simulink model "SCo3"  (Simulink 8.5)
settings: Solver=ode23t  SolverMode=SingleTasking  StartTime=0.0  StopTime=0.1  RelTol=1e-3  AbsTol=1e-3
libraries: powerlib x41, powerlib_extras x9
settings Model: Creator=azadpour  LastModifiedBy=PC  ExtModeTrigMode=oneshot  ExtModeArmWhenConnect=off  ExtModeAutoUpdateStatusClock=off
settings DataIOCC: LimitDataPoints=off
settings OptimizationCC: BlockReduction=off  BooleanDataType=off  InitFltsAndDblsToZero=on
settings DebuggingCC: SaveWithParameterizedLinksMsg=none  SignalResolutionControl=TryResolveAllWithWarning  InheritedTsInSrcMsg=none  MultiTaskDSMMsg=warning  MultiTaskCondExecSysMsg=none  FcnCallInpInsideContextMsg=UseLocalSettings  StrictBusMsg=None
settings HardwareCC: TargetUnknown=on
settings RTWCC: TemplateMakefile=grt_vc.tmf
settings GRTTargetCC: TargetFcnLib=ansi_tfl_tmw.mat

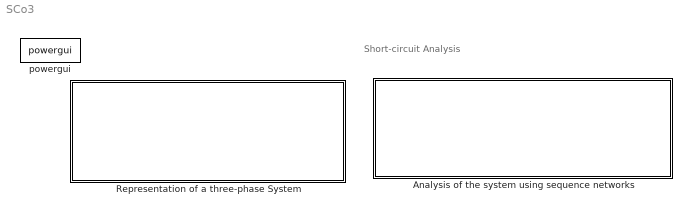
== system SCo3 ==
  note: Short-circuit Analysis
  Analysis of the system using sequence networks : Subsystem
      mask Display: disp('Analysis of the system using sequence networks')
  Representation of a three-phase System : Subsystem
      mask Display: disp('Representaton of a three-phase System')
  powergui : powerlib/powergui  SimulationMode=Continuous  SolverType=Tustin/Backward Euler (TBE)  SampleTime=0  frequency=60  SPID=off  DisableSnubberDevices=off  DisableRonSwitches=off  DisableVfSwitches=off  SwTol=0  DisplayEquations=off  Interpol=off  methode=off  Ts=0  FunctionMessages=off  echomessages=off  HookPort=off  EnableUseOfTLC=off  x0status=blocks  frequencyindice=0  Pbase=100e6  ErrMax=1e-4  Iterations=50  UnitsV=kV  UnitsW=MW  buscounter=0  RestoreLinks=warning  ResistiveCurrentMeasurement=off  Frange=[0:2:500]  Ylog=off  Xlog=on  ShowGrid=off  save=off  variable=ZData  structure=0  ZoomFFT=on  StartTime=0.0  cycles=1  DisplayStyle=1  fundamental=60  FreqAxis=off  MaxFrequency=1000  frequencyindicesteady=1  RmsSteady=1  display=off

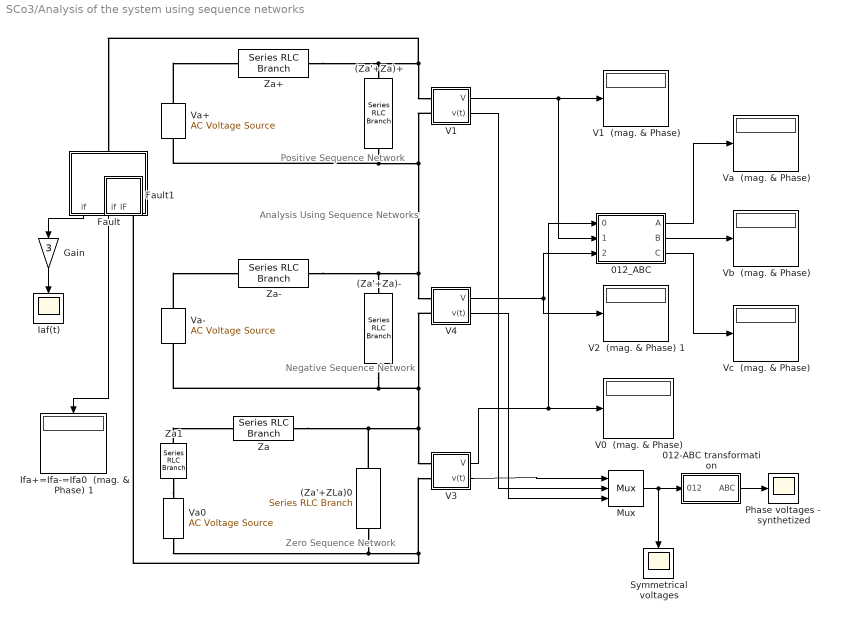
== system SCo3/Analysis of the system using sequence networks ==
  note: Positive Sequence Network
  note: Zero Sequence Network
  note: Negative Sequence Network
  note: Analysis Using
      | Sequence Networks
  (Za'+ZLa)0 : powerlib/Elements/Series RLC Branch  LConnTagsString=__new0  RConnTagsString=__new0  BranchType=RL  Resistance=0.01+0.72  Inductance=(0.05+0.54)/(2*pi*60)  SetiL0=off  InitialCurrent=0  Capacitance=1.0  Setx0=off  InitialVoltage=0  Measurements=None
  (Za'+Za)+ : powerlib/Elements/Series RLC Branch  LConnTagsString=__new0  RConnTagsString=__new0  BranchType=RL  Resistance=0.01+0.72  Inductance=(0.05+0.54)/(2*pi*60)  SetiL0=off  InitialCurrent=0  Capacitance=1.0  Setx0=off  InitialVoltage=0  Measurements=None
  (Za'+Za)- : powerlib/Elements/Series RLC Branch  LConnTagsString=__new0  RConnTagsString=__new0  BranchType=RL  Resistance=0.01+0.72  Inductance=(0.05+0.54)/(2*pi*60)  SetiL0=off  InitialCurrent=0  Capacitance=1.0  Setx0=off  InitialVoltage=0  Measurements=None
  012-ABC transformation : Subsystem
  012_ABC : Subsystem
      mask init:
      | a=cos(120*pi/180)+i*sin(120*pi/180);
      | A=[1 1 1; 1 a^2 a; 1 a a^2];
      mask Display: disp('012_ABC');
  Fault : Subsystem  mask{RF=3*0.5, time=(2.25)/60}
      mask prompts: RF "Resistance [ohm]"; time "Time [sec]"
      mask Display: plot(0,0,100,100,[40,40,57,35,51],[20,5,73,48,95],[40,51],[5,20])
  Fault1 : Subsystem  mask{RF=3*0.5, time=(2.25)/60}
      mask prompts: RF "Resistance [ohm]"; time "Time [sec]"
      mask Display: plot(0,0,100,100,[40,40,57,35,51],[20,5,73,48,95],[40,51],[5,20])
  Gain : Gain  Gain=3  SaturateOnIntegerOverflow=on  OutDataTypeStr=Inherit: Same as input  ParamDataTypeStr=Inherit: Same as input
  Iaf(t) : Scope
      settings: TickLabels=on  TimeRange=0.1  YMin=-1.5  YMax=1.5
  Ifa+=Ifa-=Ifa0  (mag. & Phase) 1 : Display
  Mux : Mux  Inputs=3
  Phase voltages -  synthetized : Scope
      settings: TickLabels=on  TimeRange=0.1  YMin=-1.3  YMax=1.3
  Symmetrical voltages : Scope
      settings: TickLabels=on  TimeRange=0.05  YMin=-1.05  YMax=1.05
  "V0  (mag. & Phase) " : Display
  V1 : Subsystem
  "V1  (mag. & Phase) " : Display
  V2  (mag. & Phase) 1 : Display
  V3 : Subsystem
  V4 : Subsystem
  "Va  (mag. & Phase) " : Display
  Va+ : powerlib/Electrical Sources/AC Voltage Source  Amplitude=1  Phase=0  Frequency=60  SampleTime=0  Measurements=None
  Va- : powerlib/Electrical Sources/AC Voltage Source  Amplitude=0  Phase=0  Frequency=60  SampleTime=0  Measurements=None
  Va0 : powerlib/Electrical Sources/AC Voltage Source  Amplitude=0  Phase=0  Frequency=60  SampleTime=0  Measurements=None
  "Vb  (mag. & Phase) " : Display
  "Vc  (mag. & Phase) " : Display
  Za : powerlib/Elements/Series RLC Branch  LConnTagsString=__new0  RConnTagsString=__new0  BranchType=RL  Resistance=0.01  Inductance=0.05/(2*pi*60)  SetiL0=off  InitialCurrent=0  Capacitance=1.0  Setx0=off  InitialVoltage=0  Measurements=None
  Za+ : powerlib/Elements/Series RLC Branch  LConnTagsString=__new0  RConnTagsString=__new0  BranchType=RL  Resistance=0.01  Inductance=0.05/(2*pi*60)  SetiL0=off  InitialCurrent=0  Capacitance=1.0  Setx0=off  InitialVoltage=0  Measurements=None
  Za- : powerlib/Elements/Series RLC Branch  LConnTagsString=__new0  RConnTagsString=__new0  BranchType=RL  Resistance=0.01  Inductance=0.05/(2*pi*60)  SetiL0=off  InitialCurrent=0  Capacitance=1.0  Setx0=off  InitialVoltage=0  Measurements=None
  Za1 : powerlib/Elements/Series RLC Branch  LConnTagsString=__new0  RConnTagsString=__new0  BranchType=Open circuit  Resistance=1  Inductance=1.0  SetiL0=off  InitialCurrent=0  Capacitance=1.0  Setx0=off  InitialVoltage=0  Measurements=None
  wires:
  Gain/1 -> Iaf(t)/1
  Fault/1(if) -> Gain/1
  Fault/2(IF) -> Ifa+=Ifa-=Ifa0  (mag. & Phase) 1/1
  012-ABC transformation/1(ABC) -> Phase voltages -  synthetized/1
  V1/2(v(t)) -> Mux/2
  V4/2(v(t)) -> Mux/3
  V3/2(v(t)) -> Mux/1
  012_ABC/1(A) -> "Va  (mag. & Phase) "/1
  012_ABC/2(B) -> "Vb  (mag. & Phase) "/1
  012_ABC/3(C) -> "Vc  (mag. & Phase) "/1
  V3/1(V) -> 012_ABC/1(0), "V0  (mag. & Phase) "/1
  V4/1(V) -> 012_ABC/3(2), V2  (mag. & Phase) 1/1
  V1/1(V) -> "V1  (mag. & Phase) "/1, 012_ABC/2(1)
  Mux/1 -> 012-ABC transformation/1(012), Symmetrical voltages/1
  connections:
  Va+/RConn1 -- Za+/LConn1
  Za-/RConn1 -- V1/LConn2 -- Va+/LConn1 -- (Za'+Za)+/RConn1 -- V4/LConn1 -- (Za'+Za)-/LConn1
  (Za'+ZLa)0/RConn1 -- Fault/RConn1 -- V3/LConn2 -- Va0/LConn1
  (Za'+ZLa)0/LConn1 -- V4/LConn2 -- Va-/LConn1 -- (Za'+Za)-/RConn1 -- V3/LConn1 -- Za/RConn1
  Va-/RConn1 -- Za-/LConn1
  Za+/RConn1 -- (Za'+Za)+/LConn1 -- V1/LConn1 -- Fault/LConn1
  Za1/RConn1 -- Va0/RConn1
  Za1/LConn1 -- Za/LConn1

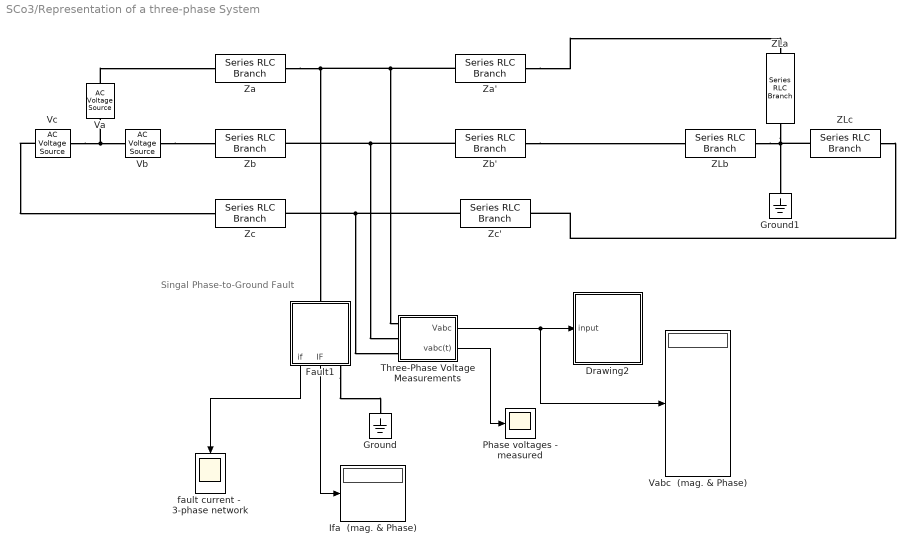
== system SCo3/Representation of a three-phase System ==
  note: Singal Phase-to-Ground Fault
  Drawing2 : Subsystem  mask(ABC and 012 Phasor Display){Bactive=off}
      mask prompts: Bactive "Block active"
      mask init:
      | global count;
      | count=0;
      mask Display: disp('Display \nabc \nand \n012\nphasors');
  Fault1 : Subsystem  mask{RF=0.5, time=(2.25)/60}
      mask prompts: RF "Resistance [ohm]"; time "Time [sec]"
      mask Display: plot(0,0,100,100,[40,40,57,35,51],[20,5,73,48,95],[40,51],[5,20])
  Ground : powerlib/Elements/Ground  LConnTagsString=a
  Ground1 : powerlib/Elements/Ground  LConnTagsString=a
  Ifa  (mag. & Phase) : Display
  Phase voltages - measured : Scope
      settings: TickLabels=on  TimeRange=0.1  YMin=-1.3  YMax=1.3
  Three-Phase Voltage Measurements : Subsystem
  Va : powerlib/Electrical Sources/AC Voltage Source  Amplitude=1  Phase=0  Frequency=60  SampleTime=0  Measurements=None
  Vabc  (mag. & Phase) : Display
  Vb : powerlib/Electrical Sources/AC Voltage Source  Amplitude=1  Phase=-120  Frequency=60  SampleTime=0  Measurements=None
  Vc : powerlib/Electrical Sources/AC Voltage Source  Amplitude=1  Phase=120  Frequency=60  SampleTime=0  Measurements=None
  ZLa : powerlib/Elements/Series RLC Branch  LConnTagsString=__new0  RConnTagsString=__new0  BranchType=RL  Resistance=0.72  Inductance=0.54/(2*pi*60)  SetiL0=off  InitialCurrent=0  Capacitance=1.0  Setx0=off  InitialVoltage=0  Measurements=None
  ZLb : powerlib/Elements/Series RLC Branch  LConnTagsString=__new0  RConnTagsString=__new0  BranchType=RL  Resistance=0.72  Inductance=0.54/(2*pi*60)  SetiL0=off  InitialCurrent=0  Capacitance=1.0  Setx0=off  InitialVoltage=0  Measurements=None
  ZLc : powerlib/Elements/Series RLC Branch  LConnTagsString=__new0  RConnTagsString=__new0  BranchType=RL  Resistance=0.72  Inductance=0.54/(2*pi*60)  SetiL0=off  InitialCurrent=0  Capacitance=1.0  Setx0=off  InitialVoltage=0  Measurements=None
  Za : powerlib/Elements/Series RLC Branch  LConnTagsString=__new0  RConnTagsString=__new0  BranchType=RL  Resistance=0.01  Inductance=0.05/(2*pi*60)  SetiL0=off  InitialCurrent=0  Capacitance=1.0  Setx0=off  InitialVoltage=0  Measurements=None
  Za' : powerlib/Elements/Series RLC Branch  LConnTagsString=__new0  RConnTagsString=__new0  BranchType=RL  Resistance=0.01  Inductance=0.05/(2*pi*60)  SetiL0=off  InitialCurrent=0  Capacitance=1.0  Setx0=off  InitialVoltage=0  Measurements=None
  Zb : powerlib/Elements/Series RLC Branch  LConnTagsString=__new0  RConnTagsString=__new0  BranchType=RL  Resistance=0.01  Inductance=0.05/(2*pi*60)  SetiL0=off  InitialCurrent=0  Capacitance=1.0  Setx0=off  InitialVoltage=0  Measurements=None
  Zb' : powerlib/Elements/Series RLC Branch  LConnTagsString=__new0  RConnTagsString=__new0  BranchType=RL  Resistance=0.01  Inductance=0.05/(2*pi*60)  SetiL0=off  InitialCurrent=0  Capacitance=1.0  Setx0=off  InitialVoltage=0  Measurements=None
  Zc : powerlib/Elements/Series RLC Branch  LConnTagsString=__new0  RConnTagsString=__new0  BranchType=RL  Resistance=0.01  Inductance=0.05/(2*pi*60)  SetiL0=off  InitialCurrent=0  Capacitance=1.0  Setx0=off  InitialVoltage=0  Measurements=None
  Zc' : powerlib/Elements/Series RLC Branch  LConnTagsString=__new0  RConnTagsString=__new0  BranchType=RL  Resistance=0.01  Inductance=0.05/(2*pi*60)  SetiL0=off  InitialCurrent=0  Capacitance=1.0  Setx0=off  InitialVoltage=0  Measurements=None
  fault current -  3-phase network : Scope
      settings: TickLabels=on  TimeRange=0.1  YMin=-1.5  YMax=1.5
  wires:
  Three-Phase Voltage Measurements/2(vabc(t)) -> Phase voltages - measured/1
  Three-Phase Voltage Measurements/1(Vabc) -> Drawing2/1(input), Vabc  (mag. & Phase)/1
  Fault1/1(if) -> fault current -  3-phase network/1
  Fault1/2(IF) -> Ifa  (mag. & Phase)/1
  connections:
  Vc/LConn1 -- Vb/LConn1 -- Va/LConn1
  Va/RConn1 -- Za/LConn1
  Vb/RConn1 -- Zb/LConn1
  Vc/RConn1 -- Zc/LConn1
  Za'/LConn1 -- Za/RConn1 -- Fault1/LConn1 -- Three-Phase Voltage Measurements/LConn1
  Zb'/LConn1 -- Zb/RConn1 -- Three-Phase Voltage Measurements/LConn2
  Zc'/LConn1 -- Zc/RConn1 -- Three-Phase Voltage Measurements/LConn3
  Fault1/RConn1 -- Ground/LConn1
  ZLa/RConn1 -- Ground1/LConn1 -- ZLc/RConn1 -- ZLb/RConn1
  Za'/RConn1 -- ZLa/LConn1
  Zb'/RConn1 -- ZLb/LConn1
  ZLc/LConn1 -- Zc'/RConn1

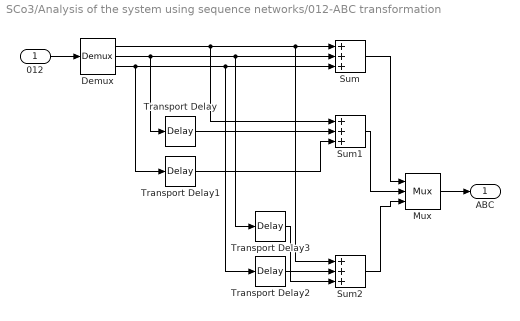
== system SCo3/Analysis of the system using sequence networks/012-ABC transformation ==
  012 : Inport
  Demux : Demux  Outputs=3
  Mux : Mux  Inputs=3
  Sum : Sum  Inputs=+++  SaturateOnIntegerOverflow=on  InputSameDT=on  OutDataTypeStr=Inherit: Same as first input
  Sum1 : Sum  Inputs=+++  SaturateOnIntegerOverflow=on  InputSameDT=on  OutDataTypeStr=Inherit: Same as first input
  Sum2 : Sum  Inputs=+++  SaturateOnIntegerOverflow=on  InputSameDT=on  OutDataTypeStr=Inherit: Same as first input
  Transport Delay : TransportDelay  DelayTime=1/(3*60)
  Transport Delay1 : TransportDelay  DelayTime=2/(3*60)
  Transport Delay2 : TransportDelay  DelayTime=1/(3*60)
  Transport Delay3 : TransportDelay  DelayTime=2/(3*60)
  ABC : Outport  InitialOutput=0
  wires:
  Transport Delay3/1 -> Sum2/2
  Transport Delay2/1 -> Sum2/3
  Transport Delay1/1 -> Sum1/3
  Transport Delay/1 -> Sum1/2
  Demux/1 -> Sum2/1, Sum/1, Sum1/1
  Demux/3 -> Transport Delay2/1, Sum/3, Transport Delay1/1
  Demux/2 -> Transport Delay3/1, Sum/2, Transport Delay/1
  Sum2/1 -> Mux/3
  Mux/1 -> ABC/1
  Sum/1 -> Mux/1
  Sum1/1 -> Mux/2
  012/1 -> Demux/1

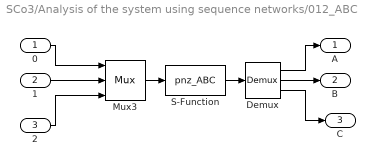
== system SCo3/Analysis of the system using sequence networks/012_ABC ==
  0 : Inport
  1 : Inport  Port=2
  2 : Inport  Port=3
  Demux : Demux  Outputs=3
  Mux3 : Mux  Inputs=3
  S-Function : S-Function  FunctionName=pnz_ABC  Parameters=A
  A : Outport  InitialOutput=0
  B : Outport  Port=2  InitialOutput=0
  C : Outport  Port=3  InitialOutput=0
  wires:
  Mux3/1 -> S-Function/1
  0/1 -> Mux3/1
  1/1 -> Mux3/2
  2/1 -> Mux3/3
  S-Function/1 -> Demux/1
  Demux/1 -> A/1
  Demux/2 -> B/1
  Demux/3 -> C/1

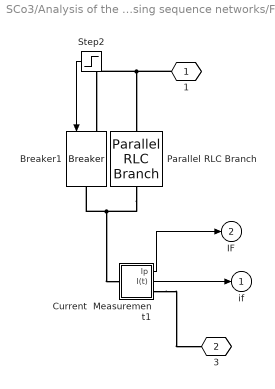
== system SCo3/Analysis of the system using sequence networks/Fault ==
  Breaker1 : powerlib/Elements/Breaker  InitialState=0  SwitchingTimes="[ 1/60  5/60 ]"  External=on  BreakerResistance=RF  SnubberResistance=1e6  SnubberCapacitance=inf  Measurements=None  MoreParameters=off  NoBreakLoop=off
  Current  Measurement1 : Subsystem
  Parallel RLC Branch : powerlib/Elements/Parallel RLC Branch  LConnTagsString=a  RConnTagsString=__new0  BranchType=R  Resistance=1e3  Inductance=1.0  SetiL0=off  InitialCurrent=0  Capacitance=1.0  Setx0=off  InitialVoltage=0  Measurements=None
  Step2 : Step  Time=time
  1 : PMIOPort  Tag=PMCPort  Port=1  Side=Left
  3 : PMIOPort  Tag=PMCPort  Port=2  Side=Right
  if : Outport  InitialOutput=0
  IF : Outport  Port=2  InitialOutput=0
  wires:
  Step2/1 -> Breaker1/1
  Current  Measurement1/2(I(t)) -> if/1
  Current  Measurement1/1(Ip) -> IF/1
  connections:
  1/RConn1 -- Breaker1/LConn1 -- Parallel RLC Branch/LConn1
  Parallel RLC Branch/RConn1 -- Breaker1/RConn1 -- Current  Measurement1/LConn1
  Current  Measurement1/RConn1 -- 3/RConn1

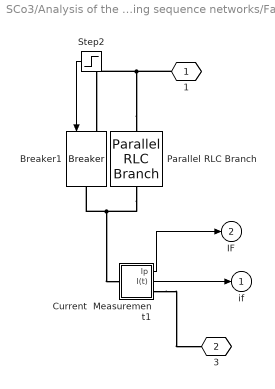
== system SCo3/Analysis of the system using sequence networks/Fault1 ==
  Breaker1 : powerlib/Elements/Breaker  InitialState=0  SwitchingTimes="[ 1/60  5/60 ]"  External=on  BreakerResistance=RF  SnubberResistance=1e6  SnubberCapacitance=inf  Measurements=None  MoreParameters=off  NoBreakLoop=off
  Current  Measurement1 : Subsystem
  Parallel RLC Branch : powerlib/Elements/Parallel RLC Branch  LConnTagsString=a  RConnTagsString=__new0  BranchType=R  Resistance=1e3  Inductance=1.0  SetiL0=off  InitialCurrent=0  Capacitance=1.0  Setx0=off  InitialVoltage=0  Measurements=None
  Step2 : Step  Time=time
  1 : PMIOPort  Tag=PMCPort  Port=1  Side=Left
  3 : PMIOPort  Tag=PMCPort  Port=2  Side=Right
  if : Outport  InitialOutput=0
  IF : Outport  Port=2  InitialOutput=0
  wires:
  Current  Measurement1/1(Ip) -> IF/1
  Current  Measurement1/2(I(t)) -> if/1
  Step2/1 -> Breaker1/1
  connections:
  Current  Measurement1/RConn1 -- 3/RConn1
  Current  Measurement1/LConn1 -- Breaker1/RConn1 -- Parallel RLC Branch/RConn1
  Parallel RLC Branch/LConn1 -- Breaker1/LConn1 -- 1/RConn1

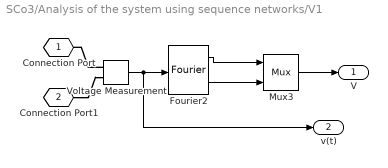
== system SCo3/Analysis of the system using sequence networks/V1 ==
  Fourier2 : powerlib_extras/Measurements/Fourier  f1=60  n=1
  Mux3 : Mux  Inputs=2
  Voltage Measurement : powerlib/Measurements/Voltage Measurement  PhasorSimulation=off  OutputType=Complex  PSBequivalent=0
  Connection Port : PMIOPort  Tag=PMCPort  Port=1  Side=Left
  Connection Port1 : PMIOPort  Tag=PMCPort  Port=2  Side=Left
  V : Outport  InitialOutput=0
  v(t) : Outport  Port=2  InitialOutput=0
  wires:
  Fourier2/1 -> Mux3/1
  Fourier2/2 -> Mux3/2
  Mux3/1 -> V/1
  Voltage Measurement/1 -> Fourier2/1, v(t)/1
  connections:
  Voltage Measurement/LConn1 -- Connection Port/RConn1
  Connection Port1/RConn1 -- Voltage Measurement/LConn2

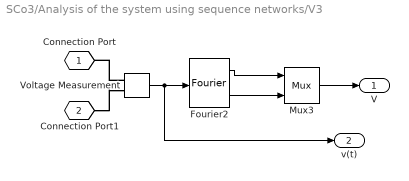
== system SCo3/Analysis of the system using sequence networks/V3 ==
  Fourier2 : powerlib_extras/Measurements/Fourier  f1=60  n=1
  Mux3 : Mux  Inputs=2
  Voltage Measurement : powerlib/Measurements/Voltage Measurement  PhasorSimulation=off  OutputType=Complex  PSBequivalent=0
  Connection Port : PMIOPort  Tag=PMCPort  Port=1  Side=Left
  Connection Port1 : PMIOPort  Tag=PMCPort  Port=2  Side=Left
  V : Outport  InitialOutput=0
  v(t) : Outport  Port=2  InitialOutput=0
  wires:
  Voltage Measurement/1 -> v(t)/1, Fourier2/1
  Mux3/1 -> V/1
  Fourier2/2 -> Mux3/2
  Fourier2/1 -> Mux3/1
  connections:
  Connection Port1/RConn1 -- Voltage Measurement/LConn2
  Voltage Measurement/LConn1 -- Connection Port/RConn1

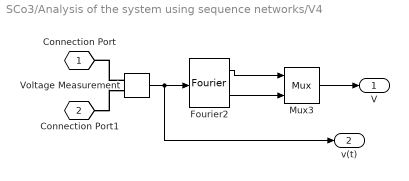
== system SCo3/Analysis of the system using sequence networks/V4 ==
  Fourier2 : powerlib_extras/Measurements/Fourier  f1=60  n=1
  Mux3 : Mux  Inputs=2
  Voltage Measurement : powerlib/Measurements/Voltage Measurement  PhasorSimulation=off  OutputType=Complex  PSBequivalent=0
  Connection Port : PMIOPort  Tag=PMCPort  Port=1  Side=Left
  Connection Port1 : PMIOPort  Tag=PMCPort  Port=2  Side=Left
  V : Outport  InitialOutput=0
  v(t) : Outport  Port=2  InitialOutput=0
  wires:
  Voltage Measurement/1 -> v(t)/1, Fourier2/1
  Mux3/1 -> V/1
  Fourier2/2 -> Mux3/2
  Fourier2/1 -> Mux3/1
  connections:
  Connection Port1/RConn1 -- Voltage Measurement/LConn2
  Voltage Measurement/LConn1 -- Connection Port/RConn1

== system SCo3/Representation of a three-phase System/Drawing2 ==
  input : Inport
  S-Function : S-Function  FunctionName=phdraw1c  Parameters=Bactive
  wires:
  input/1 -> S-Function/1

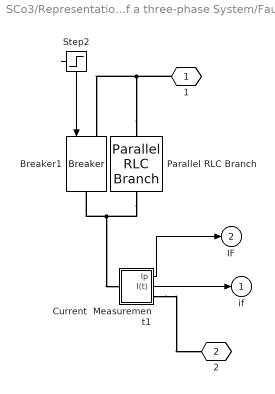
== system SCo3/Representation of a three-phase System/Fault1 ==
  Breaker1 : powerlib/Elements/Breaker  InitialState=0  SwitchingTimes="[ 1/60  5/60 ]"  External=on  BreakerResistance=RF  SnubberResistance=1e6  SnubberCapacitance=inf  Measurements=None  MoreParameters=off  NoBreakLoop=off
  Current  Measurement1 : Subsystem
  Parallel RLC Branch : powerlib/Elements/Parallel RLC Branch  LConnTagsString=a  RConnTagsString=__new0  BranchType=R  Resistance=1e3  Inductance=1.0  SetiL0=off  InitialCurrent=0  Capacitance=1.0  Setx0=off  InitialVoltage=0  Measurements=None
  Step2 : Step  Time=time
  1 : PMIOPort  Tag=PMCPort  Port=1  Side=Left
  2 : PMIOPort  Tag=PMCPort  Port=2  Side=Right
  if : Outport  InitialOutput=0
  IF : Outport  Port=2  InitialOutput=0
  wires:
  Current  Measurement1/1(Ip) -> IF/1
  Current  Measurement1/2(I(t)) -> if/1
  Step2/1 -> Breaker1/1
  connections:
  Current  Measurement1/RConn1 -- 2/RConn1
  Current  Measurement1/LConn1 -- Breaker1/RConn1 -- Parallel RLC Branch/RConn1
  Parallel RLC Branch/LConn1 -- Breaker1/LConn1 -- 1/RConn1

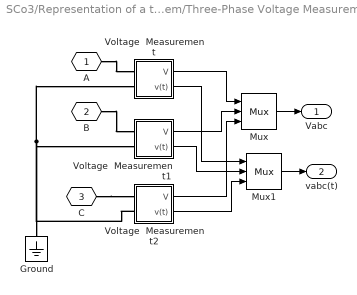
== system SCo3/Representation of a three-phase System/Three-Phase Voltage Measurements ==
  Ground : powerlib/Elements/Ground  LConnTagsString=a
  Mux : Mux  Inputs=3
  Mux1 : Mux  Inputs=3
  Voltage  Measurement : Subsystem
  Voltage  Measurement1 : Subsystem
  Voltage  Measurement2 : Subsystem
  A : PMIOPort  Tag=PMCPort  Port=1  Side=Left
  B : PMIOPort  Tag=PMCPort  Port=2  Side=Left
  C : PMIOPort  Tag=PMCPort  Port=3  Side=Left
  Vabc : Outport  InitialOutput=0
  vabc(t) : Outport  Port=2  InitialOutput=0
  wires:
  Voltage  Measurement/1(V) -> Mux/1
  Voltage  Measurement1/1(V) -> Mux/2
  Voltage  Measurement2/1(V) -> Mux/3
  Voltage  Measurement/2(v(t)) -> Mux1/1
  Voltage  Measurement1/2(v(t)) -> Mux1/2
  Voltage  Measurement2/2(v(t)) -> Mux1/3
  Mux/1 -> Vabc/1
  Mux1/1 -> vabc(t)/1
  connections:
  A/RConn1 -- Voltage  Measurement/LConn1
  B/RConn1 -- Voltage  Measurement1/LConn1
  C/RConn1 -- Voltage  Measurement2/LConn1
  Voltage  Measurement2/LConn2 -- Ground/LConn1 -- Voltage  Measurement/LConn2 -- Voltage  Measurement1/LConn2

== system SCo3/Analysis of the system using sequence networks/Fault/Current  Measurement1 ==
  Current Measurement : powerlib/Measurements/Current Measurement  PhasorSimulation=off  OutputType=Complex  PSBequivalent=0
  Fourier1 : powerlib_extras/Measurements/Fourier  f1=60  n=1
  Mux1 : Mux  Inputs=2
  + : PMIOPort  Tag=PMCPort  Port=1  Side=Left
  - : PMIOPort  Tag=PMCPort  Port=2  Side=Right
  Ip : Outport  InitialOutput=0
  I(t) : Outport  Port=2  InitialOutput=0
  wires:
  Current Measurement/1 -> Fourier1/1, I(t)/1
  Mux1/1 -> Ip/1
  Fourier1/1 -> Mux1/1
  Fourier1/2 -> Mux1/2
  connections:
  Current Measurement/LConn1 -- +/RConn1
  Current Measurement/RConn1 -- -/RConn1

== system SCo3/Analysis of the system using sequence networks/Fault1/Current  Measurement1 ==
  Current Measurement : powerlib/Measurements/Current Measurement  PhasorSimulation=off  OutputType=Complex  PSBequivalent=0
  Fourier1 : powerlib_extras/Measurements/Fourier  f1=60  n=1
  Mux1 : Mux  Inputs=2
  + : PMIOPort  Tag=PMCPort  Port=1  Side=Left
  - : PMIOPort  Tag=PMCPort  Port=2  Side=Right
  Ip : Outport  InitialOutput=0
  I(t) : Outport  Port=2  InitialOutput=0
  wires:
  Fourier1/2 -> Mux1/2
  Fourier1/1 -> Mux1/1
  Mux1/1 -> Ip/1
  Current Measurement/1 -> I(t)/1, Fourier1/1
  connections:
  Current Measurement/RConn1 -- -/RConn1
  Current Measurement/LConn1 -- +/RConn1

== system SCo3/Representation of a three-phase System/Fault1/Current  Measurement1 ==
  Current Measurement : powerlib/Measurements/Current Measurement  PhasorSimulation=off  OutputType=Complex  PSBequivalent=0
  Fourier1 : powerlib_extras/Measurements/Fourier  f1=60  n=1
  Mux1 : Mux  Inputs=2
  + : PMIOPort  Tag=PMCPort  Port=1  Side=Left
  - : PMIOPort  Tag=PMCPort  Port=2  Side=Right
  Ip : Outport  InitialOutput=0
  I(t) : Outport  Port=2  InitialOutput=0
  wires:
  Fourier1/2 -> Mux1/2
  Fourier1/1 -> Mux1/1
  Mux1/1 -> Ip/1
  Current Measurement/1 -> I(t)/1, Fourier1/1
  connections:
  Current Measurement/RConn1 -- -/RConn1
  Current Measurement/LConn1 -- +/RConn1

== system SCo3/Representation of a three-phase System/Three-Phase Voltage Measurements/Voltage  Measurement ==
  Fourier2 : powerlib_extras/Measurements/Fourier  f1=60  n=1
  Mux3 : Mux  Inputs=2
  Voltage Measurement : powerlib/Measurements/Voltage Measurement  PhasorSimulation=off  OutputType=Complex  PSBequivalent=0
  + : PMIOPort  Tag=PMCPort  Port=1  Side=Left
  - : PMIOPort  Tag=PMCPort  Port=2  Side=Left
  V : Outport  InitialOutput=0
  v(t) : Outport  Port=2  InitialOutput=0
  wires:
  Fourier2/1 -> Mux3/1
  Fourier2/2 -> Mux3/2
  Mux3/1 -> V/1
  Voltage Measurement/1 -> Fourier2/1, v(t)/1
  connections:
  -/RConn1 -- Voltage Measurement/LConn2
  +/RConn1 -- Voltage Measurement/LConn1

== system SCo3/Representation of a three-phase System/Three-Phase Voltage Measurements/Voltage  Measurement1 ==
  Fourier2 : powerlib_extras/Measurements/Fourier  f1=60  n=1
  Mux3 : Mux  Inputs=2
  Voltage Measurement : powerlib/Measurements/Voltage Measurement  PhasorSimulation=off  OutputType=Complex  PSBequivalent=0
  + : PMIOPort  Tag=PMCPort  Port=1  Side=Left
  - : PMIOPort  Tag=PMCPort  Port=2  Side=Left
  V : Outport  InitialOutput=0
  v(t) : Outport  Port=2  InitialOutput=0
  wires:
  Voltage Measurement/1 -> v(t)/1, Fourier2/1
  Mux3/1 -> V/1
  Fourier2/2 -> Mux3/2
  Fourier2/1 -> Mux3/1
  connections:
  +/RConn1 -- Voltage Measurement/LConn1
  -/RConn1 -- Voltage Measurement/LConn2

== system SCo3/Representation of a three-phase System/Three-Phase Voltage Measurements/Voltage  Measurement2 ==
  Fourier2 : powerlib_extras/Measurements/Fourier  f1=60  n=1
  Mux3 : Mux  Inputs=2
  Voltage Measurement : powerlib/Measurements/Voltage Measurement  PhasorSimulation=off  OutputType=Complex  PSBequivalent=0
  + : PMIOPort  Tag=PMCPort  Port=1  Side=Left
  - : PMIOPort  Tag=PMCPort  Port=2  Side=Left
  V : Outport  InitialOutput=0
  v(t) : Outport  Port=2  InitialOutput=0
  wires:
  Fourier2/1 -> Mux3/1
  Fourier2/2 -> Mux3/2
  Mux3/1 -> V/1
  Voltage Measurement/1 -> Fourier2/1, v(t)/1
  connections:
  -/RConn1 -- Voltage Measurement/LConn2
  +/RConn1 -- Voltage Measurement/LConn1
